simulink library "iprob"  (Simulink 8.1)
settings: Solver=ode1  StartTime=0.0  StopTime=Inf  FixedStep=0.001  RelTol=1e-3
PostLoadFcn:
  | , if any(exist('dsrtsu_mdlpostloadfcn', 'file') == [2, 3, 6]), try dsrtsu_mdlpostloadfcn('Execute', bdroot); catch fprintf('Error in PostLoadFcn (dsrtsu_mdlpostloadfcn) for model "%s":\n %s\n', bdroot, lasterr); end, end,
undefined symbols (not defined in the file or in its folder): HUNDRED_PERCENT, KIFO_ProbabTtcxThresh_s, KIFO_ProbWeigCrashPot_perc, KIFO_ProbWeigInPath_perc, KIFO_ProbWeigTtcx_perc, ZERO_FLOAT
libraries: hcu_lib x2
settings Model: DSRTSU_INTERNAL_RTI_VER=450  DSRTSU_INTERNAL_RTI_TYPE=rti1401  RTICANMMDATA=struct('GeneralSetupData',struct('modelroot','D:\PROJECTS\HAITEC\TAIWAN_HAITEC_SVN\trunk\AdasDragon\software\sw_development\arch\app\ifo','generalsettings',struct('filesettings',struct('destfolder',struct('Name','RTICANMM_FILES','Check',1),'buildfolder',struct('Name','.','Check',1),'AbsDestfolder',struct('Name','D:\PROJECTS\HAITEC\TAIWAN_HAITEC_SVN\trunk\AdasDragon\software\sw_development\arch\app\ifo\RTICANMM_FILES'),'AbsBuildfolder',struct('Name','D:\PROJECTS\HAITEC\TAIWAN_HAITEC_SVN\trunk\AdasDragon\software\sw_development\arch\app\ifo'))),'options',struct('addpaths',1,'rmpaths',1,'addtrcexclusion',logical(1),'cannavigator',struct('checkmonitoring',0),'show_usrtrc',0,'use_usrtrc',0),'advanced',struct('options',[1 1 1 1 1 1 1 1 1 1 1 1 1 1 1 1 1 1 1 1 1 1 1 1 1 1 1 1 1 1 1 1 1 1 1 1 1 1 1 1 1 1 1 1 1 1 1 1 1 1 1 1 1 1 1 1 1 1 1 1 1 1 1 1 1 1 1 1 1 1 1 1 1 1 1 1 1 1 1 1 1 1 1 1 1 1 1 1 1 1 1 1 1 1 1 1 1 1 1 1]),'MPSetup',{{}},'modelname','iprob','block','iprob'))  DSRTSU_INTERNAL_RTIFPGA=40  Creator=tescamilla  LastModifiedBy=tescamilla

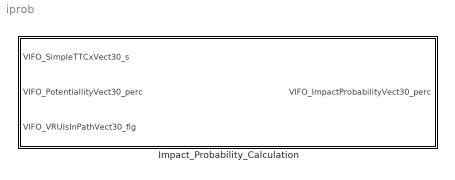
== system iprob ==
  Impact_Probability_Calculation : Subsystem

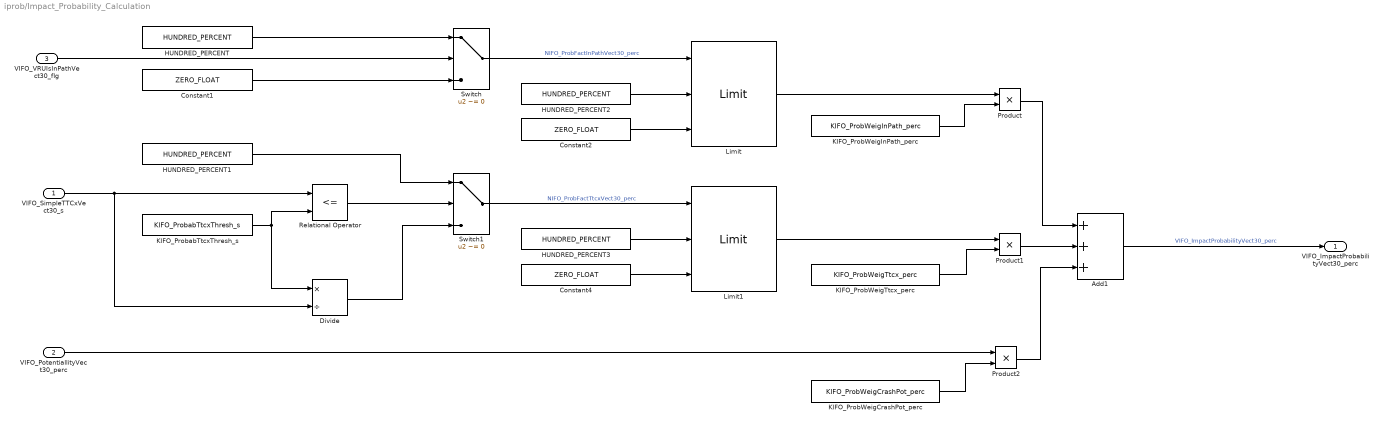
== system iprob/Impact_Probability_Calculation ==
  VIFO_SimpleTTCxVect30_s : Inport
  VIFO_PotentiallityVect30_perc : Inport  Port=2
  VIFO_VRUIsInPathVect30_flg : Inport  Port=3
  Add1 : Sum  Inputs=+++
  Constant1 : Constant  Value=ZERO_FLOAT
  Constant2 : Constant  Value=ZERO_FLOAT
  Constant4 : Constant  Value=ZERO_FLOAT
  Divide : Product  Inputs=*/
  HUNDRED_PERCENT{,1..3} (4 alike) : Constant  Value=HUNDRED_PERCENT
  KIFO_ProbWeigCrashPot_perc : Constant  Value=KIFO_ProbWeigCrashPot_perc
  KIFO_ProbWeigInPath_perc : Constant  Value=KIFO_ProbWeigInPath_perc
  KIFO_ProbWeigTtcx_perc : Constant  Value=KIFO_ProbWeigTtcx_perc
  KIFO_ProbabTtcxThresh_s : Constant  Value=KIFO_ProbabTtcxThresh_s
  Limit : hcu_lib/Limit  SystemSampleTime=-1
  Limit1 : hcu_lib/Limit  SystemSampleTime=-1
  Product : Product
  Product1 : Product
  Product2 : Product
  Relational Operator : RelationalOperator  Operator=<=  OutDataTypeStr=boolean
  Switch : Switch  Criteria=u2 ~= 0
  Switch1 : Switch  Criteria=u2 ~= 0
  VIFO_ImpactProbabilityVect30_perc : Outport
  wires:
  VIFO_VRUIsInPathVect30_flg/1 -> Switch/2
  HUNDRED_PERCENT/1 -> Switch/1
  Constant1/1 -> Switch/3
  Switch/1 -> Limit/1  "NIFO_ProbFactInPathVect30_perc"
  VIFO_SimpleTTCxVect30_s/1 -> Divide/2, Relational Operator/1
  Relational Operator/1 -> Switch1/2
  HUNDRED_PERCENT1/1 -> Switch1/1
  KIFO_ProbabTtcxThresh_s/1 -> Divide/1, Relational Operator/2
  Switch1/1 -> Limit1/1  "NIFO_ProbFactTtcxVect30_perc"
  Divide/1 -> Switch1/3
  Constant2/1 -> Limit/3
  HUNDRED_PERCENT2/1 -> Limit/2
  Constant4/1 -> Limit1/3
  Limit/1 -> Product/1
  Limit1/1 -> Product1/1
  VIFO_PotentiallityVect30_perc/1 -> Product2/1
  Product1/1 -> Add1/2
  Product/1 -> Add1/1
  Product2/1 -> Add1/3
  Add1/1 -> VIFO_ImpactProbabilityVect30_perc/1  "VIFO_ImpactProbabilityVect30_perc"
  HUNDRED_PERCENT3/1 -> Limit1/2
  KIFO_ProbWeigInPath_perc/1 -> Product/2
  KIFO_ProbWeigTtcx_perc/1 -> Product1/2
  KIFO_ProbWeigCrashPot_perc/1 -> Product2/2
